simulink model "fcsystemBechmarkold"  (R2016a)
settings: Solver=FixedStepAuto  SolverMode=MultiTasking  StartTime=0.0  StopTime=30.0  FixedStep=0.0001  MaxStep=0.0001  RelTol=1e-5
InitFcn:
  | fcsmain;
values from neighbouring files (symbols this model uses):
  C = ss1.C    [MVE.m]
  G = ss1.A    [MVE.m]
  H = ss1.B    [MVE.m]
  K1 = Ktemp(1)    [MVE.m]
  K2 = Ktemp(2:end)    [MVE.m]
  Ke = acker(G',C',P)'    [MVE.m]
  Ts = 0.1    [MVE.m]
undefined symbols (not defined in the file or in its folder): alliedsignaleff, beta0, beta1, beta2, cm_kt, cm_kv, cm_maxtorque, cm_R, Cp, cp_inertia, dc, faradays, fc_activearea, fc_anode_volume, fc_cathode_volume, fc_inlet_flow_constant, fc_numberofcells, fc_outlet_flow_constant, fcx0, gamma, hydrogengasconstant, hydrogenmolarmass, im_volume, membranedrydensity, membranedryeqvweight, membranethickness, nitrogengasconstant, nitrogenmolarmass, om_At, om_Cd, om_outlet_choke_pr, om_volume, oxygengasconstant, oxygenmolarmass, phimax0, phimax1, phimax2, phimax3, phimax4, psimax0, psimax1, psimax2, psimax3, psimax4, psimax5, R, rho, Ta, universalgasconstant, vaporgasconstant, vapormolarmass
libraries: simulink x1
(part 3 of 3)

== system fcsystemBechmarkold/Fuel Cell Stack System/Stack/Cathode Mass Flow Model/Outlet Flow Properties to O2, N2 and Vapor Mass Flow ==
  note: Units
      | Pressure - Pascal, bar
      | Temperature - Kelvin
      | Voltage - Volt
      | Current - Ampere
      | Mass Flow - kg/sec
      | Rotational Speed - rad/sec
      | Power - Watt
      | humidity or relative humidity - 0 to 1
  Air Flow out : Inport
  1 - Total Mass Flow 2 - Temperature 3 - Pressure 4 - Relative Humidity 5 - Oxygen Mole Fraction (in Dry Air) : Demux  Outputs=5
  Constant1 : Constant  Value=vapormolarmass
  Constant2 : Constant
  Constant3 : Constant
  Dry Air Molar Mass : Fcn  Expr=u*oxygenmolarmass+(1-u)*nitrogenmolarmass
  Mole Fraction to Mass Fraction : Fcn  Expr=(u*oxygenmolarmass)/(u*oxygenmolarmass+(1-u)*nitrogenmolarmass)
  Product{2,6,8..9} (4 alike) : Product  SaturateOnIntegerOverflow=on  InputSameDT=on  OutDataTypeStr=Inherit: Same as first input
  Product4 : Product  Inputs=*/  SaturateOnIntegerOverflow=on  InputSameDT=on  OutDataTypeStr=Inherit: Same as first input
  Product5 : Product  Inputs=*/  SaturateOnIntegerOverflow=on  InputSameDT=on  OutDataTypeStr=Inherit: Same as first input
  Product7 : Product  Inputs=*/  SaturateOnIntegerOverflow=on  InputSameDT=on  OutDataTypeStr=Inherit: Same as first input
  Saturation Pressure (Pa) : Subsystem
  Sum4 : Sum  Inputs=-|+  SaturateOnIntegerOverflow=on  InputSameDT=on  OutDataTypeStr=Inherit: Same as first input
  Sum5 : Sum  Inputs=++|  SaturateOnIntegerOverflow=on  InputSameDT=on  OutDataTypeStr=Inherit: Same as first input
  Sum6 : Sum  Inputs=-+|  SaturateOnIntegerOverflow=on  InputSameDT=on  OutDataTypeStr=Inherit: Same as first input
  Sum7 : Sum  Inputs=-|+  SaturateOnIntegerOverflow=on  InputSameDT=on  OutDataTypeStr=Inherit: Same as first input
  Vapor Mass Flow out : Outport
  Oxygen Mass Flow out : Outport  Port=2
  Nitrogen Mass Flow out : Outport  Port=3
  wires:
  Product9/1 -> Nitrogen Mass Flow out/1  "Nitrogen Mass Flow"
  Sum7/1 -> Product9/2
  Constant3/1 -> Sum7/2
  Mole Fraction to Mass Fraction/1 -> Sum7/1, Product8/2  "Oxygen Mass Fraction"
  Product8/1 -> Oxygen Mass Flow out/1  "Oxygen Mass Flow"
  Product7/1 -> Product9/1, Product8/1, Sum6/1  "dry air mass flow"
  1 - Total Mass Flow 2 - Temperature 3 - Pressure 4 - Relative Humidity 5 - Oxygen Mole Fraction (in Dry Air)/5 -> Mole Fraction to Mass Fraction/1, Dry Air Molar Mass/1
  Sum6/1 -> Vapor Mass Flow out/1  "vapor mass flow"
  1 - Total Mass Flow 2 - Temperature 3 - Pressure 4 - Relative Humidity 5 - Oxygen Mole Fraction (in Dry Air)/1 -> Sum6/2, Product7/1
  Constant2/1 -> Sum5/1
  Product6/1 -> Sum5/2  "Humidity Ratio"
  Sum5/1 -> Product7/2
  Product5/1 -> Product6/1
  Product2/1 -> Product5/1, Sum4/1  "vapor partial pressure"
  Sum4/1 -> Product5/2  "dry air partial pressure"
  1 - Total Mass Flow 2 - Temperature 3 - Pressure 4 - Relative Humidity 5 - Oxygen Mole Fraction (in Dry Air)/4 -> Product2/2
  Saturation Pressure (Pa)/1(Saturation Pressure (Pa)) -> Product2/1
  Product4/1 -> Product6/2
  Constant1/1 -> Product4/1
  Dry Air Molar Mass/1 -> Product4/2
  1 - Total Mass Flow 2 - Temperature 3 - Pressure 4 - Relative Humidity 5 - Oxygen Mole Fraction (in Dry Air)/3 -> Sum4/2
  1 - Total Mass Flow 2 - Temperature 3 - Pressure 4 - Relative Humidity 5 - Oxygen Mole Fraction (in Dry Air)/2 -> Saturation Pressure (Pa)/1(Temperature (K))
  Air Flow out/1 -> 1 - Total Mass Flow 2 - Temperature 3 - Pressure 4 - Relative Humidity 5 - Oxygen Mole Fraction (in Dry Air)/1

== system fcsystemBechmarkold/Fuel Cell Stack System/Stack/Cathode Mass Flow Model/Oxygen Balance ==
  O2 Mass Flow In (kg/s) : Inport
  O2 Mass Flow out (kg/s) : Inport  Port=2
  O2 Mass reacted (kg/s) : Inport  Port=3
  FC Temperature (K) : Inport  Port=4
  Initial Condition (kg) : Constant  Value=fcx0(1)
  Integrator : Integrator  InitialConditionSource=external
  Mux : Mux  Inputs=2
  Partial Pressure : Fcn  Expr=u[1]*oxygengasconstant*u[2]/fc_cathode_volume
  Sum : Sum  Inputs=+--  SaturateOnIntegerOverflow=on  InputSameDT=on  OutDataTypeStr=Inherit: Same as first input
  O2 Mass (kg) : Outport
  O2 Partial Pressure : Outport  Port=2
  tag scope: mO2=global
  wires:
  O2 Mass Flow In (kg/s)/1 -> Sum/1
  O2 Mass Flow out (kg/s)/1 -> Sum/2
  O2 Mass reacted (kg/s)/1 -> Sum/3
  Sum/1 -> Integrator/1
  Initial Condition (kg)/1 -> Integrator/2
  FC Temperature (K)/1 -> Mux/2
  Integrator/1 -> O2 Mass (kg)/1, Mux/1, [mO2]
  Mux/1 -> Partial Pressure/1
  Partial Pressure/1 -> O2 Partial Pressure/1

== system fcsystemBechmarkold/Fuel Cell Stack System/Stack/Cathode Mass Flow Model/Pressure Calculation ==
  O2 Partial Pressure : Inport
  N2 Partial Pressure : Inport  Port=2
  Vapor Partial Pressure : Inport  Port=3
  Product : Product  Inputs=*/  SaturateOnIntegerOverflow=on  InputSameDT=on  OutDataTypeStr=Inherit: Same as first input
  Sum : Sum  Inputs=+|+  SaturateOnIntegerOverflow=on  InputSameDT=on  OutDataTypeStr=Inherit: Same as first input
  Sum1 : Sum  Inputs=+|+  SaturateOnIntegerOverflow=on  InputSameDT=on  OutDataTypeStr=Inherit: Same as first input
  Cathode Pressure : Outport
  O2 Mole Fraction : Outport  Port=2
  wires:
  N2 Partial Pressure/1 -> Sum/2
  O2 Partial Pressure/1 -> Sum/1, Product/1
  Product/1 -> O2 Mole Fraction/1  "O2 Mole Fraction"
  Sum/1 -> Product/2, Sum1/1  "Dry Air Partial Pressure"
  Vapor Partial Pressure/1 -> Sum1/2
  Sum1/1 -> Cathode Pressure/1  "Total Pressure"

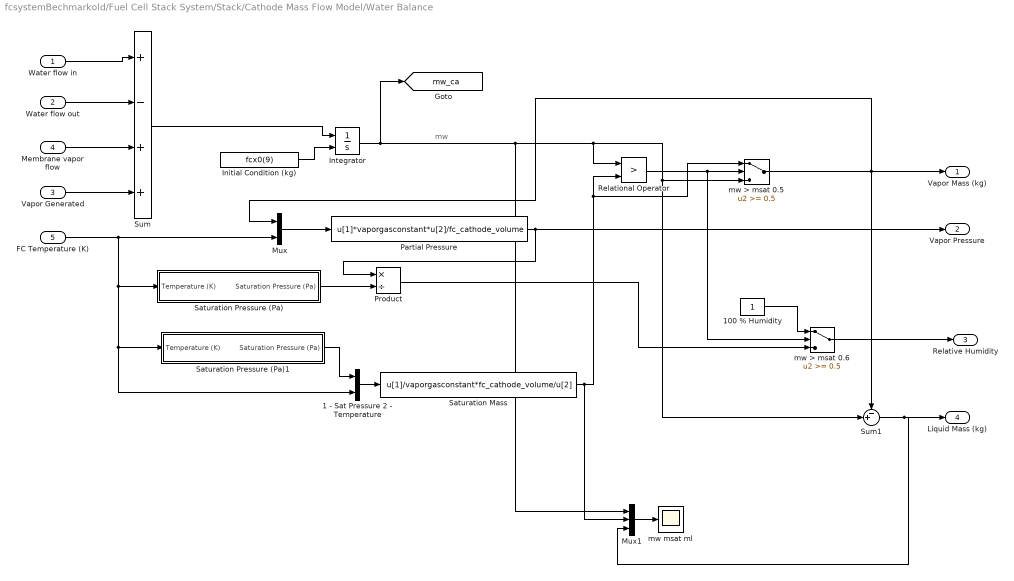
== system fcsystemBechmarkold/Fuel Cell Stack System/Stack/Cathode Mass Flow Model/Water Balance ==
  note: mw
  Water flow in : Inport
  Water flow out : Inport  Port=2
  Vapor Generated : Inport  Port=3
  Membrane vapor flow : Inport  Port=4
  FC Temperature (K) : Inport  Port=5
  1 - Sat Pressure 2 - Temperature : Mux  Inputs=2
  100 % Humidity : Constant
  Initial Condition (kg) : Constant  Value=fcx0(9)
  Integrator : Integrator  InitialConditionSource=external
  Mux : Mux  Inputs=2
  Mux1 : Mux  Inputs=3
  Partial Pressure : Fcn  Expr=u[1]*vaporgasconstant*u[2]/fc_cathode_volume
  Product : Product  Inputs=*/  SaturateOnIntegerOverflow=on  InputSameDT=on  OutDataTypeStr=Inherit: Same as first input
  Relational Operator : RelationalOperator  Operator=>  InputSameDT=on
  Saturation Mass : Fcn  Expr=u[1]/vaporgasconstant*fc_cathode_volume/u[2]
  Saturation Pressure (Pa) : Subsystem
  Saturation Pressure (Pa)1 : Subsystem
  Sum : Sum  Inputs=+-++  SaturateOnIntegerOverflow=on  InputSameDT=on  OutDataTypeStr=Inherit: Same as first input
  Sum1 : Sum  Inputs=-+|  SaturateOnIntegerOverflow=on  InputSameDT=on  OutDataTypeStr=Inherit: Same as first input
  mw msat ml : Scope
  mw > msat 0.5 : Switch  Threshold=0.5  SaturateOnIntegerOverflow=on  InputSameDT=on
  mw > msat 0.6 : Switch  Threshold=0.5  SaturateOnIntegerOverflow=on  InputSameDT=on
  Vapor Mass (kg) : Outport
  Vapor Pressure : Outport  Port=2
  Relative Humidity : Outport  Port=3
  Liquid Mass (kg) : Outport  Port=4
  tag scope: mw_ca=global
  wires:
  Water flow in/1 -> Sum/1
  Water flow out/1 -> Sum/2
  Membrane vapor flow/1 -> Sum/3
  FC Temperature (K)/1 -> Mux/2, Saturation Pressure (Pa)/1(Temperature (K)), 1 - Sat Pressure 2 - Temperature/2, Saturation Pressure (Pa)1/1(Temperature (K))
  Integrator/1 -> [mw_ca], Relational Operator/1, mw > msat 0.5/3, Sum1/2, Mux1/1
  Initial Condition (kg)/1 -> Integrator/2
  Saturation Pressure (Pa)/1(Saturation Pressure (Pa)) -> Product/2
  Partial Pressure/1 -> Product/1, Vapor Pressure/1
  Mux/1 -> Partial Pressure/1
  Saturation Pressure (Pa)1/1(Saturation Pressure (Pa)) -> 1 - Sat Pressure 2 - Temperature/1
  1 - Sat Pressure 2 - Temperature/1 -> Saturation Mass/1
  Saturation Mass/1 -> Relational Operator/2, mw > msat 0.5/1, Mux1/2
  100 % Humidity/1 -> mw > msat 0.6/1
  Product/1 -> mw > msat 0.6/3
  mw > msat 0.6/1 -> Relative Humidity/1
  mw > msat 0.5/1 -> Mux/1, Sum1/1, Vapor Mass (kg)/1
  Relational Operator/1 -> mw > msat 0.5/2, mw > msat 0.6/2
  Sum1/1 -> Liquid Mass (kg)/1, Mux1/3
  Sum/1 -> Integrator/1
  Vapor Generated/1 -> Sum/4
  Mux1/1 -> mw msat ml/1

== system fcsystemBechmarkold/Fuel Cell Stack System/Stack/Stack Voltage Model/Saturation Pressure (Pa) ==
  Temperature (K) : Inport
  333.15K : Switch  Threshold=333.15  SaturateOnIntegerOverflow=on  InputSameDT=on
  433.15K : Switch  Threshold=433.15  SaturateOnIntegerOverflow=on  InputSameDT=on
  533.15K : Switch  SaturateOnIntegerOverflow=on  InputSameDT=on
  Water Sat. Pressure in kPa (using 4th order approx) 333.15K<t<433.15K : Fcn  Expr=1.508306069874139e-006*u^4-0.00184416225407*u^3+0.85777718452468*u^2-1.796665242102233e+002*u+1.428163901107325e+004
  Water Sat. Pressure in kPa (using 4th order approx) 433.15<t<533.15 : Fcn  Expr=1.338811201296496e-006*u^4-0.00154136533415*u^3+0.65477998701526*u^2-1.191331991860853e+002*u+7.506492157825003e+003
  Water Sat. Pressure in kPa (using 4th order approx) t<333.15K : Fcn  Expr=6.853193243616891e-007*u^4-7.432459524835483e-004*u^3+0.30413751828818*u^2-55.61363113326989*u+3.831800671740628e+003
  Water Sat. Pressure in kPa (using 4th order approx) t>533.15K : Fcn  Expr=1.648503329422670e-6*u^4-0.00209262218193*u^3+1.01793196387371*u^2-2.241752317908023e2*u+1.878246444328017e4
  kPa to Pa : Gain  Gain=1000  SaturateOnIntegerOverflow=on  OutDataTypeStr=Inherit: Same as input  ParamDataTypeStr=Inherit: Same as input
  Saturation Pressure (Pa) : Outport
  wires:
  Temperature (K)/1 -> Water Sat. Pressure in kPa (using 4th order approx) t>533.15K/1, Water Sat. Pressure in kPa (using 4th order approx) 433.15<t<533.15/1, Water Sat. Pressure in kPa (using 4th order approx) 333.15K<t<433.15K/1, Water Sat. Pressure in kPa (using 4th order approx) t<333.15K/1, 533.15K/2, 433.15K/2, 333.15K/2
  533.15K/1 -> kPa to Pa/1
  kPa to Pa/1 -> Saturation Pressure (Pa)/1
  433.15K/1 -> 533.15K/3
  Water Sat. Pressure in kPa (using 4th order approx) t>533.15K/1 -> 533.15K/1
  Water Sat. Pressure in kPa (using 4th order approx) 433.15<t<533.15/1 -> 433.15K/1
  333.15K/1 -> 433.15K/3
  Water Sat. Pressure in kPa (using 4th order approx) 333.15K<t<433.15K/1 -> 333.15K/1
  Water Sat. Pressure in kPa (using 4th order approx) t<333.15K/1 -> 333.15K/3

== system fcsystemBechmarkold/Fuel Cell Stack System/Compressor/Compressor/Calculate Humidity Change/Saturation Pressure (Pa) ==
  Temperature (K) : Inport
  333.15K : Switch  Threshold=333.15  SaturateOnIntegerOverflow=on  InputSameDT=on
  433.15K : Switch  Threshold=433.15  SaturateOnIntegerOverflow=on  InputSameDT=on
  533.15K : Switch  Threshold=533.15  SaturateOnIntegerOverflow=on  InputSameDT=on
  Water Sat. Pressure in kPa (using 4th order approx) 333.15K<t<433.15K : Fcn  Expr=1.508306069874139e-006*u^4-0.00184416225407*u^3+0.85777718452468*u^2-1.796665242102233e+002*u+1.428163901107325e+004
  Water Sat. Pressure in kPa (using 4th order approx) 433.15<t<533.15 : Fcn  Expr=1.338811201296496e-006*u^4-0.00154136533415*u^3+0.65477998701526*u^2-1.191331991860853e+002*u+7.506492157825003e+003
  Water Sat. Pressure in kPa (using 4th order approx) t<333.15K : Fcn  Expr=6.853193243616891e-007*u^4-7.432459524835483e-004*u^3+0.30413751828818*u^2-55.61363113326989*u+3.831800671740628e+003
  Water Sat. Pressure in kPa (using 4th order approx) t>533.15K : Fcn  Expr=1.648503329422670e-6*u^4-0.00209262218193*u^3+1.01793196387371*u^2-2.241752317908023e2*u+1.878246444328017e4
  kPa to Pa : Gain  Gain=1000  SaturateOnIntegerOverflow=on  OutDataTypeStr=Inherit: Same as input  ParamDataTypeStr=Inherit: Same as input
  Saturation Pressure (Pa) : Outport
  wires:
  Water Sat. Pressure in kPa (using 4th order approx) t<333.15K/1 -> 333.15K/3
  Water Sat. Pressure in kPa (using 4th order approx) 333.15K<t<433.15K/1 -> 333.15K/1
  333.15K/1 -> 433.15K/3
  Water Sat. Pressure in kPa (using 4th order approx) 433.15<t<533.15/1 -> 433.15K/1
  Water Sat. Pressure in kPa (using 4th order approx) t>533.15K/1 -> 533.15K/1
  433.15K/1 -> 533.15K/3
  kPa to Pa/1 -> Saturation Pressure (Pa)/1
  533.15K/1 -> kPa to Pa/1
  Temperature (K)/1 -> 333.15K/2, 433.15K/2, 533.15K/2, Water Sat. Pressure in kPa (using 4th order approx) t<333.15K/1, Water Sat. Pressure in kPa (using 4th order approx) 333.15K<t<433.15K/1, Water Sat. Pressure in kPa (using 4th order approx) 433.15<t<533.15/1, Water Sat. Pressure in kPa (using 4th order approx) t>533.15K/1

== system fcsystemBechmarkold/Fuel Cell Stack System/Compressor/Compressor/Calculate Humidity Change/Saturation Pressure (Pa)1 ==
  Temperature (K) : Inport
  333.15K : Switch  Threshold=333.15  SaturateOnIntegerOverflow=on  InputSameDT=on
  433.15K : Switch  Threshold=433.15  SaturateOnIntegerOverflow=on  InputSameDT=on
  533.15K : Switch  Threshold=533.15  SaturateOnIntegerOverflow=on  InputSameDT=on
  Display{1..5} (5 alike) : Display
  Water Sat. Pressure in kPa (using 4th order approx) 333.15K<t<433.15K : Fcn  Expr=1.508306069874139e-006*u^4-0.00184416225407*u^3+0.85777718452468*u^2-1.796665242102233e+002*u+1.428163901107325e+004
  Water Sat. Pressure in kPa (using 4th order approx) 433.15<t<533.15 : Fcn  Expr=1.338811201296496e-006*u^4-0.00154136533415*u^3+0.65477998701526*u^2-1.191331991860853e+002*u+7.506492157825003e+003
  Water Sat. Pressure in kPa (using 4th order approx) t<333.15K : Fcn  Expr=6.853193243616891e-007*u^4-7.432459524835483e-004*u^3+0.30413751828818*u^2-55.61363113326989*u+3.831800671740628e+003
  Water Sat. Pressure in kPa (using 4th order approx) t>533.15K : Fcn  Expr=1.648503329422670e-6*u^4-0.00209262218193*u^3+1.01793196387371*u^2-2.241752317908023e2*u+1.878246444328017e4
  kPa to Pa : Gain  Gain=1000  SaturateOnIntegerOverflow=on  OutDataTypeStr=Inherit: Same as input  ParamDataTypeStr=Inherit: Same as input
  Saturation Pressure (Pa) : Outport
  wires:
  kPa to Pa/1 -> Saturation Pressure (Pa)/1
  Water Sat. Pressure in kPa (using 4th order approx) t>533.15K/1 -> 533.15K/1
  Water Sat. Pressure in kPa (using 4th order approx) 433.15<t<533.15/1 -> 433.15K/1
  Water Sat. Pressure in kPa (using 4th order approx) 333.15K<t<433.15K/1 -> 333.15K/1
  333.15K/1 -> 433.15K/3, Display1/1
  433.15K/1 -> 533.15K/3, Display2/1
  Water Sat. Pressure in kPa (using 4th order approx) t<333.15K/1 -> 333.15K/3, Display3/1
  533.15K/1 -> kPa to Pa/1, Display4/1
  Temperature (K)/1 -> Water Sat. Pressure in kPa (using 4th order approx) t>533.15K/1, Water Sat. Pressure in kPa (using 4th order approx) 433.15<t<533.15/1, Water Sat. Pressure in kPa (using 4th order approx) 333.15K<t<433.15K/1, Water Sat. Pressure in kPa (using 4th order approx) t<333.15K/1, 533.15K/2, 433.15K/2, 333.15K/2, Display5/1

== system fcsystemBechmarkold/Fuel Cell Stack System/Compressor/Compressor/Compressor  Map/Compressor Efficiency ==
  Flow lb/min : Inport
  Pressure Ratio : Inport  Port=2
  Look-Up Table (2-D) : Lookup2D  RowIndex=alliedsignalflow  ColumnIndex=alliedsignalpr  Table=alliedsignaleff  SaturateOnIntegerOverflow=on  InputSameDT=on
  Efficiency : Outport
  wires:
  Look-Up Table (2-D)/1 -> Efficiency/1
  Pressure Ratio/1 -> Look-Up Table (2-D)/2
  Flow lb/min/1 -> Look-Up Table (2-D)/1

== system fcsystemBechmarkold/Fuel Cell Stack System/Compressor/Compressor/Compressor  Map/Jensen&Kristensen Compressor Map ==
  note: SAE 1999-01-0908
  Pressure Ratio : Inport
  Corrected Speed (rpm) : Inport  Port=2
  1 Phi 2 Uc : Mux  Inputs=2
  "1 Psi 2 phimax 3 beta 4 psimax " : Mux
  Flowkg : Fcn  Expr=u[1]*rho*pi/4*dc*dc*u[2]
  Ma : Fcn  Expr=u/sqrt(gamma*R*Ta)
  Mux : Mux  Inputs=2
  Phi : Fcn  Expr=u[2]*(1-exp(u[3]*(u[1]/u[4]-1)))
  Psi : Fcn  Expr=Cp*Ta*(u[1]^((gamma-1)/gamma)-1)/0.5/u[2]/u[2]
  Uc : Fcn  Expr=pi*dc*u/60
  beta : Fcn  Expr=beta2*u^2+beta1*u+beta0
  phimax : Fcn  Expr=phimax4*u^4+phimax3*u^3+phimax2*u^2+phimax1*u+phimax0
  psimax : Fcn  Expr=psimax5*u^5+psimax4*u^4+psimax3*u^3+psimax2*u^2+psimax1*u+psimax0
  Air Flow (kg/sec) : Outport
  wires:
  Psi/1 -> "1 Psi 2 phimax 3 beta 4 psimax "/1
  psimax/1 -> "1 Psi 2 phimax 3 beta 4 psimax "/4
  "1 Psi 2 phimax 3 beta 4 psimax "/1 -> Phi/1
  Phi/1 -> 1 Phi 2 Uc/1
  beta/1 -> "1 Psi 2 phimax 3 beta 4 psimax "/3
  phimax/1 -> "1 Psi 2 phimax 3 beta 4 psimax "/2
  Flowkg/1 -> Air Flow (kg/sec)/1
  1 Phi 2 Uc/1 -> Flowkg/1
  Ma/1 -> phimax/1, beta/1, psimax/1
  Mux/1 -> Psi/1
  Uc/1 -> 1 Phi 2 Uc/2, Mux/2, Ma/1
  Pressure Ratio/1 -> Mux/1
  Corrected Speed (rpm)/1 -> Uc/1

== system fcsystemBechmarkold/Fuel Cell Stack System/Stack/Anode Mass Flow Model/Water Balance/Saturation Pressure (Pa) ==
  Temperature (K) : Inport
  333.15K : Switch  Threshold=333.15  SaturateOnIntegerOverflow=on  InputSameDT=on
  433.15K : Switch  Threshold=433.15  SaturateOnIntegerOverflow=on  InputSameDT=on
  533.15K : Switch  Threshold=533.15  SaturateOnIntegerOverflow=on  InputSameDT=on
  Water Sat. Pressure in kPa (using 4th order approx) 333.15K<t<433.15K : Fcn  Expr=1.508306069874139e-006*u^4-0.00184416225407*u^3+0.85777718452468*u^2-1.796665242102233e+002*u+1.428163901107325e+004
  Water Sat. Pressure in kPa (using 4th order approx) 433.15<t<533.15 : Fcn  Expr=1.338811201296496e-006*u^4-0.00154136533415*u^3+0.65477998701526*u^2-1.191331991860853e+002*u+7.506492157825003e+003
  Water Sat. Pressure in kPa (using 4th order approx) t<333.15K : Fcn  Expr=6.853193243616891e-007*u^4-7.432459524835483e-004*u^3+0.30413751828818*u^2-55.61363113326989*u+3.831800671740628e+003
  Water Sat. Pressure in kPa (using 4th order approx) t>533.15K : Fcn  Expr=1.648503329422670e-6*u^4-0.00209262218193*u^3+1.01793196387371*u^2-2.241752317908023e2*u+1.878246444328017e4
  kPa to Pa : Gain  Gain=1000  SaturateOnIntegerOverflow=on  OutDataTypeStr=Inherit: Same as input  ParamDataTypeStr=Inherit: Same as input
  Saturation Pressure (Pa) : Outport
  wires:
  Temperature (K)/1 -> Water Sat. Pressure in kPa (using 4th order approx) t>533.15K/1, Water Sat. Pressure in kPa (using 4th order approx) 433.15<t<533.15/1, Water Sat. Pressure in kPa (using 4th order approx) 333.15K<t<433.15K/1, Water Sat. Pressure in kPa (using 4th order approx) t<333.15K/1, 533.15K/2, 433.15K/2, 333.15K/2
  533.15K/1 -> kPa to Pa/1
  kPa to Pa/1 -> Saturation Pressure (Pa)/1
  433.15K/1 -> 533.15K/3
  Water Sat. Pressure in kPa (using 4th order approx) t>533.15K/1 -> 533.15K/1
  Water Sat. Pressure in kPa (using 4th order approx) 433.15<t<533.15/1 -> 433.15K/1
  333.15K/1 -> 433.15K/3
  Water Sat. Pressure in kPa (using 4th order approx) 333.15K<t<433.15K/1 -> 333.15K/1
  Water Sat. Pressure in kPa (using 4th order approx) t<333.15K/1 -> 333.15K/3

== system fcsystemBechmarkold/Fuel Cell Stack System/Stack/Anode Mass Flow Model/Water Balance/Saturation Pressure (Pa)1 ==
  Temperature (K) : Inport
  333.15K : Switch  Threshold=333.15  SaturateOnIntegerOverflow=on  InputSameDT=on
  433.15K : Switch  Threshold=433.15  SaturateOnIntegerOverflow=on  InputSameDT=on
  533.15K : Switch  Threshold=533.15  SaturateOnIntegerOverflow=on  InputSameDT=on
  Water Sat. Pressure in kPa (using 4th order approx) 333.15K<t<433.15K : Fcn  Expr=1.508306069874139e-006*u^4-0.00184416225407*u^3+0.85777718452468*u^2-1.796665242102233e+002*u+1.428163901107325e+004
  Water Sat. Pressure in kPa (using 4th order approx) 433.15<t<533.15 : Fcn  Expr=1.338811201296496e-006*u^4-0.00154136533415*u^3+0.65477998701526*u^2-1.191331991860853e+002*u+7.506492157825003e+003
  Water Sat. Pressure in kPa (using 4th order approx) t<333.15K : Fcn  Expr=6.853193243616891e-007*u^4-7.432459524835483e-004*u^3+0.30413751828818*u^2-55.61363113326989*u+3.831800671740628e+003
  Water Sat. Pressure in kPa (using 4th order approx) t>533.15K : Fcn  Expr=1.648503329422670e-6*u^4-0.00209262218193*u^3+1.01793196387371*u^2-2.241752317908023e2*u+1.878246444328017e4
  kPa to Pa : Gain  Gain=1000  SaturateOnIntegerOverflow=on  OutDataTypeStr=Inherit: Same as input  ParamDataTypeStr=Inherit: Same as input
  Saturation Pressure (Pa) : Outport
  wires:
  Water Sat. Pressure in kPa (using 4th order approx) t<333.15K/1 -> 333.15K/3
  Water Sat. Pressure in kPa (using 4th order approx) 333.15K<t<433.15K/1 -> 333.15K/1
  333.15K/1 -> 433.15K/3
  Water Sat. Pressure in kPa (using 4th order approx) 433.15<t<533.15/1 -> 433.15K/1
  Water Sat. Pressure in kPa (using 4th order approx) t>533.15K/1 -> 533.15K/1
  433.15K/1 -> 533.15K/3
  kPa to Pa/1 -> Saturation Pressure (Pa)/1
  533.15K/1 -> kPa to Pa/1
  Temperature (K)/1 -> 333.15K/2, 433.15K/2, 533.15K/2, Water Sat. Pressure in kPa (using 4th order approx) t<333.15K/1, Water Sat. Pressure in kPa (using 4th order approx) 333.15K<t<433.15K/1, Water Sat. Pressure in kPa (using 4th order approx) 433.15<t<533.15/1, Water Sat. Pressure in kPa (using 4th order approx) t>533.15K/1

== system fcsystemBechmarkold/Fuel Cell Stack System/Stack/Anode Mass Flow Model/inlet flow properties to mass flow/Saturation Pressure (Pa) ==
  Temperature (K) : Inport
  333.15K : Switch  Threshold=333.15  SaturateOnIntegerOverflow=on  InputSameDT=on
  433.15K : Switch  Threshold=433.15  SaturateOnIntegerOverflow=on  InputSameDT=on
  533.15K : Switch  Threshold=533.15  SaturateOnIntegerOverflow=on  InputSameDT=on
  Water Sat. Pressure in kPa (using 4th order approx) 333.15K<t<433.15K : Fcn  Expr=1.508306069874139e-006*u^4-0.00184416225407*u^3+0.85777718452468*u^2-1.796665242102233e+002*u+1.428163901107325e+004
  Water Sat. Pressure in kPa (using 4th order approx) 433.15<t<533.15 : Fcn  Expr=1.338811201296496e-006*u^4-0.00154136533415*u^3+0.65477998701526*u^2-1.191331991860853e+002*u+7.506492157825003e+003
  Water Sat. Pressure in kPa (using 4th order approx) t<333.15K : Fcn  Expr=6.853193243616891e-007*u^4-7.432459524835483e-004*u^3+0.30413751828818*u^2-55.61363113326989*u+3.831800671740628e+003
  Water Sat. Pressure in kPa (using 4th order approx) t>533.15K : Fcn  Expr=1.648503329422670e-6*u^4-0.00209262218193*u^3+1.01793196387371*u^2-2.241752317908023e2*u+1.878246444328017e4
  kPa to Pa : Gain  Gain=1000  SaturateOnIntegerOverflow=on  OutDataTypeStr=Inherit: Same as input  ParamDataTypeStr=Inherit: Same as input
  Saturation Pressure (Pa) : Outport
  wires:
  Temperature (K)/1 -> Water Sat. Pressure in kPa (using 4th order approx) t>533.15K/1, Water Sat. Pressure in kPa (using 4th order approx) 433.15<t<533.15/1, Water Sat. Pressure in kPa (using 4th order approx) 333.15K<t<433.15K/1, Water Sat. Pressure in kPa (using 4th order approx) t<333.15K/1, 533.15K/2, 433.15K/2, 333.15K/2
  533.15K/1 -> kPa to Pa/1
  kPa to Pa/1 -> Saturation Pressure (Pa)/1
  433.15K/1 -> 533.15K/3
  Water Sat. Pressure in kPa (using 4th order approx) t>533.15K/1 -> 533.15K/1
  Water Sat. Pressure in kPa (using 4th order approx) 433.15<t<533.15/1 -> 433.15K/1
  333.15K/1 -> 433.15K/3
  Water Sat. Pressure in kPa (using 4th order approx) 333.15K<t<433.15K/1 -> 333.15K/1
  Water Sat. Pressure in kPa (using 4th order approx) t<333.15K/1 -> 333.15K/3

== system fcsystemBechmarkold/Fuel Cell Stack System/Stack/Anode Mass Flow Model/outlet flow properties to mass flow/Saturation Pressure (Pa) ==
  Temperature (K) : Inport
  333.15K : Switch  Threshold=333.15  SaturateOnIntegerOverflow=on  InputSameDT=on
  433.15K : Switch  Threshold=433.15  SaturateOnIntegerOverflow=on  InputSameDT=on
  533.15K : Switch  Threshold=533.15  SaturateOnIntegerOverflow=on  InputSameDT=on
  Water Sat. Pressure in kPa (using 4th order approx) 333.15K<t<433.15K : Fcn  Expr=1.508306069874139e-006*u^4-0.00184416225407*u^3+0.85777718452468*u^2-1.796665242102233e+002*u+1.428163901107325e+004
  Water Sat. Pressure in kPa (using 4th order approx) 433.15<t<533.15 : Fcn  Expr=1.338811201296496e-006*u^4-0.00154136533415*u^3+0.65477998701526*u^2-1.191331991860853e+002*u+7.506492157825003e+003
  Water Sat. Pressure in kPa (using 4th order approx) t<333.15K : Fcn  Expr=6.853193243616891e-007*u^4-7.432459524835483e-004*u^3+0.30413751828818*u^2-55.61363113326989*u+3.831800671740628e+003
  Water Sat. Pressure in kPa (using 4th order approx) t>533.15K : Fcn  Expr=1.648503329422670e-6*u^4-0.00209262218193*u^3+1.01793196387371*u^2-2.241752317908023e2*u+1.878246444328017e4
  kPa to Pa : Gain  Gain=1000  SaturateOnIntegerOverflow=on  OutDataTypeStr=Inherit: Same as input  ParamDataTypeStr=Inherit: Same as input
  Saturation Pressure (Pa) : Outport
  wires:
  Temperature (K)/1 -> Water Sat. Pressure in kPa (using 4th order approx) t>533.15K/1, Water Sat. Pressure in kPa (using 4th order approx) 433.15<t<533.15/1, Water Sat. Pressure in kPa (using 4th order approx) 333.15K<t<433.15K/1, Water Sat. Pressure in kPa (using 4th order approx) t<333.15K/1, 533.15K/2, 433.15K/2, 333.15K/2
  533.15K/1 -> kPa to Pa/1
  kPa to Pa/1 -> Saturation Pressure (Pa)/1
  433.15K/1 -> 533.15K/3
  Water Sat. Pressure in kPa (using 4th order approx) t>533.15K/1 -> 533.15K/1
  Water Sat. Pressure in kPa (using 4th order approx) 433.15<t<533.15/1 -> 433.15K/1
  333.15K/1 -> 433.15K/3
  Water Sat. Pressure in kPa (using 4th order approx) 333.15K<t<433.15K/1 -> 333.15K/1
  Water Sat. Pressure in kPa (using 4th order approx) t<333.15K/1 -> 333.15K/3

== system fcsystemBechmarkold/Fuel Cell Stack System/Stack/Cathode Mass Flow Model/Inlet Flow Properties to O2, N2 and Vapor Mass Flow/Saturation Pressure (Pa) ==
  Temperature (K) : Inport
  333.15K : Switch  Threshold=333.15  SaturateOnIntegerOverflow=on  InputSameDT=on
  433.15K : Switch  Threshold=433.15  SaturateOnIntegerOverflow=on  InputSameDT=on
  533.15K : Switch  Threshold=533.15  SaturateOnIntegerOverflow=on  InputSameDT=on
  Water Sat. Pressure in kPa (using 4th order approx) 333.15K<t<433.15K : Fcn  Expr=1.508306069874139e-006*u^4-0.00184416225407*u^3+0.85777718452468*u^2-1.796665242102233e+002*u+1.428163901107325e+004
  Water Sat. Pressure in kPa (using 4th order approx) 433.15<t<533.15 : Fcn  Expr=1.338811201296496e-006*u^4-0.00154136533415*u^3+0.65477998701526*u^2-1.191331991860853e+002*u+7.506492157825003e+003
  Water Sat. Pressure in kPa (using 4th order approx) t<333.15K : Fcn  Expr=6.853193243616891e-007*u^4-7.432459524835483e-004*u^3+0.30413751828818*u^2-55.61363113326989*u+3.831800671740628e+003
  Water Sat. Pressure in kPa (using 4th order approx) t>533.15K : Fcn  Expr=1.648503329422670e-6*u^4-0.00209262218193*u^3+1.01793196387371*u^2-2.241752317908023e2*u+1.878246444328017e4
  kPa to Pa : Gain  Gain=1000  SaturateOnIntegerOverflow=on  OutDataTypeStr=Inherit: Same as input  ParamDataTypeStr=Inherit: Same as input
  Saturation Pressure (Pa) : Outport
  wires:
  Temperature (K)/1 -> Water Sat. Pressure in kPa (using 4th order approx) t>533.15K/1, Water Sat. Pressure in kPa (using 4th order approx) 433.15<t<533.15/1, Water Sat. Pressure in kPa (using 4th order approx) 333.15K<t<433.15K/1, Water Sat. Pressure in kPa (using 4th order approx) t<333.15K/1, 533.15K/2, 433.15K/2, 333.15K/2
  533.15K/1 -> kPa to Pa/1
  kPa to Pa/1 -> Saturation Pressure (Pa)/1
  433.15K/1 -> 533.15K/3
  Water Sat. Pressure in kPa (using 4th order approx) t>533.15K/1 -> 533.15K/1
  Water Sat. Pressure in kPa (using 4th order approx) 433.15<t<533.15/1 -> 433.15K/1
  333.15K/1 -> 433.15K/3
  Water Sat. Pressure in kPa (using 4th order approx) 333.15K<t<433.15K/1 -> 333.15K/1
  Water Sat. Pressure in kPa (using 4th order approx) t<333.15K/1 -> 333.15K/3

== system fcsystemBechmarkold/Fuel Cell Stack System/Stack/Cathode Mass Flow Model/Outlet Flow Properties to O2, N2 and Vapor Mass Flow/Saturation Pressure (Pa) ==
  Temperature (K) : Inport
  333.15K : Switch  Threshold=333.15  SaturateOnIntegerOverflow=on  InputSameDT=on
  433.15K : Switch  Threshold=433.15  SaturateOnIntegerOverflow=on  InputSameDT=on
  533.15K : Switch  Threshold=533.15  SaturateOnIntegerOverflow=on  InputSameDT=on
  Water Sat. Pressure in kPa (using 4th order approx) 333.15K<t<433.15K : Fcn  Expr=1.508306069874139e-006*u^4-0.00184416225407*u^3+0.85777718452468*u^2-1.796665242102233e+002*u+1.428163901107325e+004
  Water Sat. Pressure in kPa (using 4th order approx) 433.15<t<533.15 : Fcn  Expr=1.338811201296496e-006*u^4-0.00154136533415*u^3+0.65477998701526*u^2-1.191331991860853e+002*u+7.506492157825003e+003
  Water Sat. Pressure in kPa (using 4th order approx) t<333.15K : Fcn  Expr=6.853193243616891e-007*u^4-7.432459524835483e-004*u^3+0.30413751828818*u^2-55.61363113326989*u+3.831800671740628e+003
  Water Sat. Pressure in kPa (using 4th order approx) t>533.15K : Fcn  Expr=1.648503329422670e-6*u^4-0.00209262218193*u^3+1.01793196387371*u^2-2.241752317908023e2*u+1.878246444328017e4
  kPa to Pa : Gain  Gain=1000  SaturateOnIntegerOverflow=on  OutDataTypeStr=Inherit: Same as input  ParamDataTypeStr=Inherit: Same as input
  Saturation Pressure (Pa) : Outport
  wires:
  Temperature (K)/1 -> Water Sat. Pressure in kPa (using 4th order approx) t>533.15K/1, Water Sat. Pressure in kPa (using 4th order approx) 433.15<t<533.15/1, Water Sat. Pressure in kPa (using 4th order approx) 333.15K<t<433.15K/1, Water Sat. Pressure in kPa (using 4th order approx) t<333.15K/1, 533.15K/2, 433.15K/2, 333.15K/2
  533.15K/1 -> kPa to Pa/1
  kPa to Pa/1 -> Saturation Pressure (Pa)/1
  433.15K/1 -> 533.15K/3
  Water Sat. Pressure in kPa (using 4th order approx) t>533.15K/1 -> 533.15K/1
  Water Sat. Pressure in kPa (using 4th order approx) 433.15<t<533.15/1 -> 433.15K/1
  333.15K/1 -> 433.15K/3
  Water Sat. Pressure in kPa (using 4th order approx) 333.15K<t<433.15K/1 -> 333.15K/1
  Water Sat. Pressure in kPa (using 4th order approx) t<333.15K/1 -> 333.15K/3

== system fcsystemBechmarkold/Fuel Cell Stack System/Stack/Cathode Mass Flow Model/Water Balance/Saturation Pressure (Pa) ==
  Temperature (K) : Inport
  333.15K : Switch  Threshold=333.15  SaturateOnIntegerOverflow=on  InputSameDT=on
  433.15K : Switch  Threshold=433.15  SaturateOnIntegerOverflow=on  InputSameDT=on
  533.15K : Switch  Threshold=533.15  SaturateOnIntegerOverflow=on  InputSameDT=on
  Water Sat. Pressure in kPa (using 4th order approx) 333.15K<t<433.15K : Fcn  Expr=1.508306069874139e-006*u^4-0.00184416225407*u^3+0.85777718452468*u^2-1.796665242102233e+002*u+1.428163901107325e+004
  Water Sat. Pressure in kPa (using 4th order approx) 433.15<t<533.15 : Fcn  Expr=1.338811201296496e-006*u^4-0.00154136533415*u^3+0.65477998701526*u^2-1.191331991860853e+002*u+7.506492157825003e+003
  Water Sat. Pressure in kPa (using 4th order approx) t<333.15K : Fcn  Expr=6.853193243616891e-007*u^4-7.432459524835483e-004*u^3+0.30413751828818*u^2-55.61363113326989*u+3.831800671740628e+003
  Water Sat. Pressure in kPa (using 4th order approx) t>533.15K : Fcn  Expr=1.648503329422670e-6*u^4-0.00209262218193*u^3+1.01793196387371*u^2-2.241752317908023e2*u+1.878246444328017e4
  kPa to Pa : Gain  Gain=1000  SaturateOnIntegerOverflow=on  OutDataTypeStr=Inherit: Same as input  ParamDataTypeStr=Inherit: Same as input
  Saturation Pressure (Pa) : Outport
  wires:
  Temperature (K)/1 -> Water Sat. Pressure in kPa (using 4th order approx) t>533.15K/1, Water Sat. Pressure in kPa (using 4th order approx) 433.15<t<533.15/1, Water Sat. Pressure in kPa (using 4th order approx) 333.15K<t<433.15K/1, Water Sat. Pressure in kPa (using 4th order approx) t<333.15K/1, 533.15K/2, 433.15K/2, 333.15K/2
  533.15K/1 -> kPa to Pa/1
  kPa to Pa/1 -> Saturation Pressure (Pa)/1
  433.15K/1 -> 533.15K/3
  Water Sat. Pressure in kPa (using 4th order approx) t>533.15K/1 -> 533.15K/1
  Water Sat. Pressure in kPa (using 4th order approx) 433.15<t<533.15/1 -> 433.15K/1
  333.15K/1 -> 433.15K/3
  Water Sat. Pressure in kPa (using 4th order approx) 333.15K<t<433.15K/1 -> 333.15K/1
  Water Sat. Pressure in kPa (using 4th order approx) t<333.15K/1 -> 333.15K/3

== system fcsystemBechmarkold/Fuel Cell Stack System/Stack/Cathode Mass Flow Model/Water Balance/Saturation Pressure (Pa)1 ==
  Temperature (K) : Inport
  333.15K : Switch  Threshold=333.15  SaturateOnIntegerOverflow=on  InputSameDT=on
  433.15K : Switch  Threshold=433.15  SaturateOnIntegerOverflow=on  InputSameDT=on
  533.15K : Switch  Threshold=533.15  SaturateOnIntegerOverflow=on  InputSameDT=on
  Water Sat. Pressure in kPa (using 4th order approx) 333.15K<t<433.15K : Fcn  Expr=1.508306069874139e-006*u^4-0.00184416225407*u^3+0.85777718452468*u^2-1.796665242102233e+002*u+1.428163901107325e+004
  Water Sat. Pressure in kPa (using 4th order approx) 433.15<t<533.15 : Fcn  Expr=1.338811201296496e-006*u^4-0.00154136533415*u^3+0.65477998701526*u^2-1.191331991860853e+002*u+7.506492157825003e+003
  Water Sat. Pressure in kPa (using 4th order approx) t<333.15K : Fcn  Expr=6.853193243616891e-007*u^4-7.432459524835483e-004*u^3+0.30413751828818*u^2-55.61363113326989*u+3.831800671740628e+003
  Water Sat. Pressure in kPa (using 4th order approx) t>533.15K : Fcn  Expr=1.648503329422670e-6*u^4-0.00209262218193*u^3+1.01793196387371*u^2-2.241752317908023e2*u+1.878246444328017e4
  kPa to Pa : Gain  Gain=1000  SaturateOnIntegerOverflow=on  OutDataTypeStr=Inherit: Same as input  ParamDataTypeStr=Inherit: Same as input
  Saturation Pressure (Pa) : Outport
  wires:
  Temperature (K)/1 -> Water Sat. Pressure in kPa (using 4th order approx) t>533.15K/1, Water Sat. Pressure in kPa (using 4th order approx) 433.15<t<533.15/1, Water Sat. Pressure in kPa (using 4th order approx) 333.15K<t<433.15K/1, Water Sat. Pressure in kPa (using 4th order approx) t<333.15K/1, 533.15K/2, 433.15K/2, 333.15K/2
  533.15K/1 -> kPa to Pa/1
  kPa to Pa/1 -> Saturation Pressure (Pa)/1
  433.15K/1 -> 533.15K/3
  Water Sat. Pressure in kPa (using 4th order approx) t>533.15K/1 -> 533.15K/1
  Water Sat. Pressure in kPa (using 4th order approx) 433.15<t<533.15/1 -> 433.15K/1
  333.15K/1 -> 433.15K/3
  Water Sat. Pressure in kPa (using 4th order approx) 333.15K<t<433.15K/1 -> 333.15K/1
  Water Sat. Pressure in kPa (using 4th order approx) t<333.15K/1 -> 333.15K/3
